simulink model "CustomClockRxModel"  (R2026a)
settings: Solver=FixedStepDiscrete  StopTime=100000
libraries: hdlsllib x6
settings Model: DataTypeOverride=Off  Creator=jiemingx  LastModifiedBy=jiemingx
settings OptimizationCC: ConditionallyExecuteInputs=off  InheritOutputTypeSmallerThanSingle=on
settings DebuggingCC: ArtificialAlgebraicLoopMsg=error  MergeDetectMultiDrivingBlocksExec=error  SingleTaskRateTransMsg=error
settings HardwareCC: ProdHWDeviceType=ASIC/FPGA->ASIC/FPGA  TargetBitPerLong=64.0  TargetBitPerPointer=64.0  TargetBitPerSizeT=64.0  TargetBitPerPtrDiffT=64.0  TargetLongLongMode=on  TargetIntDivRoundTo=Zero  TargetEndianess=LittleEndian  TargetWordSize=64.0  TargetHWDeviceType=Custom Processor->MATLAB Host Computer  ProdEqTarget=off
settings ModelReferenceCC: PropagateSignalLabelsOutOfModel=on

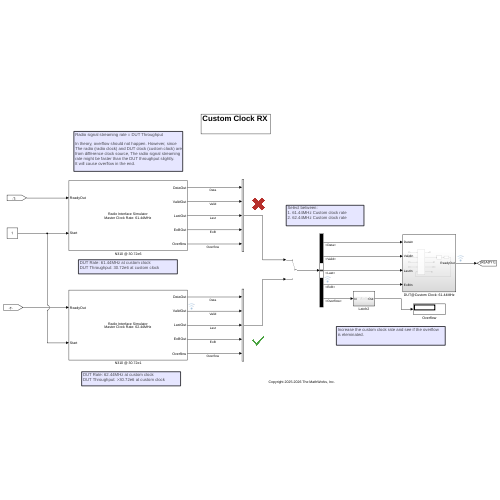
[thumbnail: Simulink's stored preview of the top-level diagram]
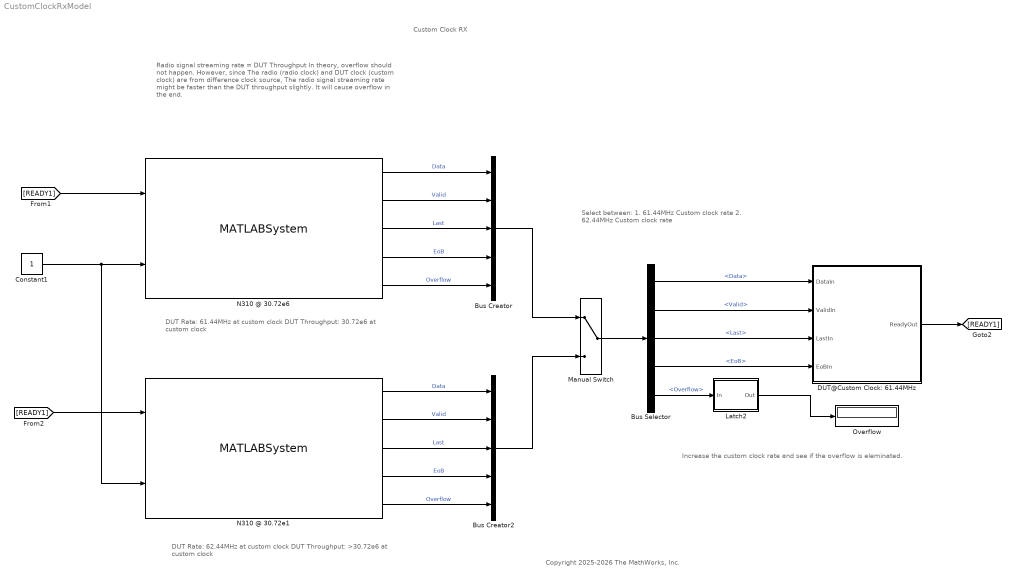
== system CustomClockRxModel ==
  note: DUT Rate: 61.44MHz at custom clock
      | DUT Throughput: 30.72e6 at custom clock
  note: Radio signal streaming rate = DUT Throughput
      |
      | In theory, overflow should not happen. However, since
      | The radio (radio clock) and DUT clock (custom clock) are
      | from difference clock source, The radio signal streaming
      | rate might be faster than the DUT throughput slightly.
      | It will cause overflow in the end.
  note: Custom Clock RX
  note: Increase the custom clock rate and see if the overflow
      | is eleminated.
  note: Select between:
      | 1. 61.44MHz Custom clock rate
      | 2. 62.44MHz Custom clock rate
  note: DUT Rate: 62.44MHz at custom clock
      | DUT Throughput: >30.72e6 at custom clock
  note: Copyright 2025-2026 The MathWorks, Inc.
  Bus Creator : BusCreator  Inputs=5
  Bus Creator2 : BusCreator  Inputs=5
  Bus Selector : BusSelector  OutputSignals=Data,Valid,Last,EoB,Overflow
  Constant1 : Constant  OutDataTypeStr=boolean  SampleTime=1
  DUT@Custom Clock: 61.44MHz : Subsystem
  Latch2 : Subsystem
  Manual Switch : ManualSwitch
  N310 @ 30.72e1 : MATLABSystem  System=RadioInterfaceSim  Device=N310  TXRX=RX  ClockSource=Custom  SampleRate=61.44e6/2  DUTClockRate=62.44e6  InputDataSource=[1:10000]  SimulateUsing=Interpreted execution  ClockUncertainty=on  Uncertainty=1  Jitter=-20
      mask Type: RadioInterfaceSim
  N310 @ 30.72e6 : MATLABSystem  System=RadioInterfaceSim  Device=N310  TXRX=RX  ClockSource=Custom  SampleRate=61.44e6/2  DUTClockRate=61.44e6  InputDataSource=[1:10000]  SimulateUsing=Interpreted execution  ClockUncertainty=on  Uncertainty=1  Jitter=-20
      mask Type: RadioInterfaceSim
  Overflow : Display
  wires:
  [READY1] -> N310 @ 30.72e6/1
  Latch2/1(Out) -> Overflow/1
  Constant1/1 -> N310 @ 30.72e1/2, N310 @ 30.72e6/2
  DUT@Custom Clock: 61.44MHz/1(ReadyOut) -> [READY1]
  Bus Selector/3 -> DUT@Custom Clock: 61.44MHz/3(LastIn)  "<Last>"
  Bus Creator/1 -> Manual Switch/1
  N310 @ 30.72e6/2 -> Bus Creator/2  "Valid"
  Bus Selector/1 -> DUT@Custom Clock: 61.44MHz/1(DataIn)  "<Data>"
  N310 @ 30.72e6/1 -> Bus Creator/1  "Data"
  Bus Selector/2 -> DUT@Custom Clock: 61.44MHz/2(ValidIn)  "<Valid>"
  Manual Switch/1 -> Bus Selector/1
  N310 @ 30.72e6/3 -> Bus Creator/3  "Last"
  N310 @ 30.72e6/4 -> Bus Creator/4  "EoB"
  Bus Selector/4 -> DUT@Custom Clock: 61.44MHz/4(EoBIn)  "<EoB>"
  N310 @ 30.72e6/5 -> Bus Creator/5  "Overflow"
  N310 @ 30.72e1/3 -> Bus Creator2/3  "Last"
  N310 @ 30.72e1/1 -> Bus Creator2/1  "Data"
  N310 @ 30.72e1/5 -> Bus Creator2/5  "Overflow"
  N310 @ 30.72e1/4 -> Bus Creator2/4  "EoB"
  N310 @ 30.72e1/2 -> Bus Creator2/2  "Valid"
  Bus Creator2/1 -> Manual Switch/2
  Bus Selector/5 -> Latch2/1(In)  "<Overflow>"
  [READY1] -> N310 @ 30.72e1/1

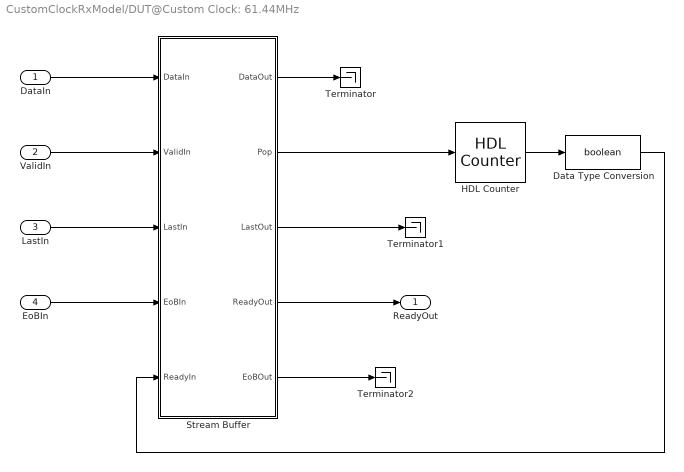
== system CustomClockRxModel/DUT@Custom Clock: 61.44MHz ==
  DataIn : Inport
  ValidIn : Inport  Port=2
  LastIn : Inport  Port=3
  EoBIn : Inport  Port=4
  Data Type Conversion : DataTypeConversion  OutDataTypeStr=boolean  SaturateOnIntegerOverflow=off  RndMeth=Floor
  HDL Counter : hdlsllib/Sources/HDL Counter  CountType=Free running  CountInit=0  CountStep=1  CountMax=25  CountFromType=Initial value  CountFrom=0  CountResetPort=off  CountLoadPort=off  CountEnbPort=on  CountDirPort=off  CountHitOutputPort=off  CountDataType=Unsigned  CountWordLen=1  CountFracLen=0  CountSampTime=1
  Stream Buffer : Subsystem
  Terminator : Terminator
  Terminator1 : Terminator
  Terminator2 : Terminator
  ReadyOut : Outport
  wires:
  HDL Counter/1 -> Data Type Conversion/1
  ValidIn/1 -> Stream Buffer/2(ValidIn)
  Data Type Conversion/1 -> Stream Buffer/5(ReadyIn)
  DataIn/1 -> Stream Buffer/1(DataIn)
  LastIn/1 -> Stream Buffer/3(LastIn)
  Stream Buffer/1(DataOut) -> Terminator/1
  Stream Buffer/2(Pop) -> HDL Counter/1
  Stream Buffer/3(LastOut) -> Terminator1/1
  Stream Buffer/4(ReadyOut) -> ReadyOut/1
  Stream Buffer/5(EoBOut) -> Terminator2/1
  EoBIn/1 -> Stream Buffer/4(EoBIn)

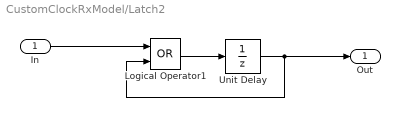
== system CustomClockRxModel/Latch2 ==
  In : Inport
  Logical Operator1 : Logic  Operator=OR  AllPortsSameDT=off  OutDataTypeStr=boolean
  Unit Delay : UnitDelay  SampleTime=-1
  Out : Outport
  wires:
  Unit Delay/1 -> Out/1, Logical Operator1/2
  In/1 -> Logical Operator1/1
  Logical Operator1/1 -> Unit Delay/1

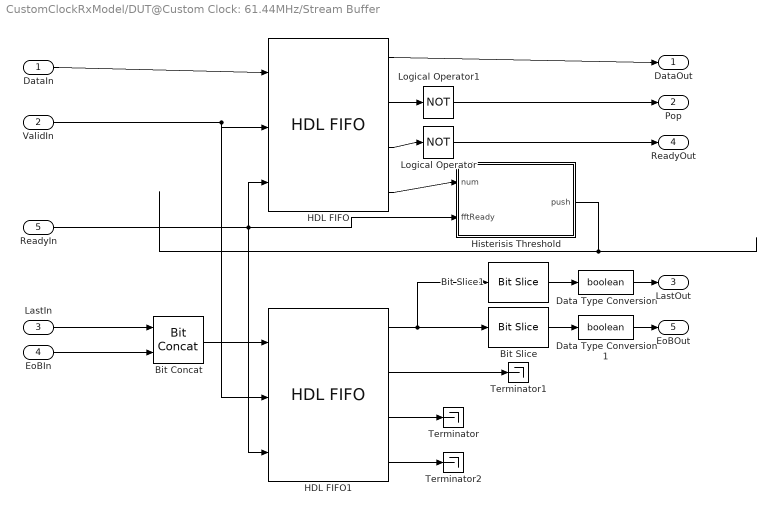
== system CustomClockRxModel/DUT@Custom Clock: 61.44MHz/Stream Buffer ==
  DataIn : Inport
  ValidIn : Inport  Port=2
  LastIn : Inport  Port=3
  EoBIn : Inport  Port=4
  ReadyIn : Inport  Port=5
  Bit Concat : hdlsllib/Logic and Bit Operations/Bit Concat  numInputs=2
  Bit Slice : hdlsllib/Logic and Bit Operations/Bit Slice  lidx=0  ridx=0
  Bit Slice1 : hdlsllib/Logic and Bit Operations/Bit Slice  lidx=1  ridx=1
  Data Type Conversion : DataTypeConversion  OutDataTypeStr=boolean  SaturateOnIntegerOverflow=off  RndMeth=Floor
  Data Type Conversion1 : DataTypeConversion  OutDataTypeStr=boolean  SaturateOnIntegerOverflow=off  RndMeth=Floor
  HDL FIFO : hdlsllib/HDL RAMs/HDL FIFO  fifo_size=512  mode=Classic  ratio=1  dataDim=1  push_msg=Warning  pop_msg=Warning  show_empty=on  show_full=on  show_num=on  LabelModeActiveChoice_Mode=Classic  rst_port=off
  HDL FIFO1 : hdlsllib/HDL RAMs/HDL FIFO  fifo_size=512  mode=Classic  ratio=1  dataDim=1  push_msg=Warning  pop_msg=Warning  show_empty=on  show_full=on  show_num=on  LabelModeActiveChoice_Mode=Classic  rst_port=off
  Histerisis Threshold : MATLAB Function  TreatAsAtomicUnit=on
  Logical Operator : Logic  Operator=NOT  AllPortsSameDT=off  OutDataTypeStr=boolean
  Logical Operator1 : Logic  Operator=NOT  AllPortsSameDT=off  OutDataTypeStr=boolean
  Terminator : Terminator
  Terminator1 : Terminator
  Terminator2 : Terminator
  DataOut : Outport
  Pop : Outport  Port=2
  LastOut : Outport  Port=3
  ReadyOut : Outport  Port=4
  EoBOut : Outport  Port=5
  wires:
  Logical Operator/1 -> ReadyOut/1
  HDL FIFO/4 -> Histerisis Threshold/1(num)
  HDL FIFO/2 -> Logical Operator1/1
  Histerisis Threshold/1(push) -> ?
  DataIn/1 -> HDL FIFO/1
  HDL FIFO/1 -> DataOut/1
  HDL FIFO/3 -> Logical Operator/1
  ValidIn/1 -> HDL FIFO1/2, HDL FIFO/2
  ReadyIn/1 -> HDL FIFO1/3, HDL FIFO/3, Histerisis Threshold/2(fftReady)
  HDL FIFO1/3 -> Terminator/1
  HDL FIFO1/4 -> Terminator2/1
  HDL FIFO1/2 -> Terminator1/1
  HDL FIFO1/1 -> Bit Slice1/1, Bit Slice/1
  LastIn/1 -> Bit Concat/1
  EoBIn/1 -> Bit Concat/2
  Bit Concat/1 -> HDL FIFO1/1
  Bit Slice1/1 -> Data Type Conversion/1
  Bit Slice/1 -> Data Type Conversion1/1
  Data Type Conversion/1 -> LastOut/1
  Data Type Conversion1/1 -> EoBOut/1
  Logical Operator1/1 -> Pop/1

== matlab function CustomClockRxModel/DUT@Custom Clock: 61.44MHz/Stream Buffer/Histerisis Threshold ==
  data: num input; push output; fftReady input boolean
function push = fcn(num, fftReady)

persistent state;
THRESHOLD0 = 0;
THRESHOLD1 = 1024;

if isempty(state)
    state = false;
end

if(state)
    if(fftReady)
        push = true;
    else
        push = false;
    end
else
    push = false;
end

if(num >= THRESHOLD1 && ~state)
    state = true;
elseif(num == THRESHOLD0 || ~fftReady)
    state = false;
end
